simulink model "Ninad_deshpande_Suspensionmodel"  (R2024b)
settings: Solver=ode45  StartTime=0.0  StopTime=10  RelTol=1e-3  EnableMultiTasking=on
values from neighbouring files (symbols this model uses):
  a = 400    [Ninad_deshpande_suspensionscript.m]
  b = 2.5e3    (= 2500)    [Ninad_deshpande_suspensionscript.m]
  Ks = 20e3    (= 20000)    [Ninad_deshpande_suspensionscript.m]
  M_u = 50    [Ninad_deshpande_suspensionscript.m]
settings Model: Creator=lenovo  LastModifiedBy=lenovo
settings SolverCC: AlgebraicLoopSolver=TrustRegion
settings DataIOCC: LimitDataPoints=on  SaveFormat=Array  ReturnWorkspaceOutputs=off
settings OptimizationCC: LifeSpan=inf
settings DebuggingCC: UnconnectedInputMsg=warning  UnconnectedOutputMsg=warning  UnconnectedLineMsg=warning  SFUnexpectedBacktrackingDiag=warning  SFNoUnconditionalDefaultTransitionDiag=warning  SFExecutionAtInitializationDiag=none  ArithmeticOperatorsInVariantConditions=warning
settings HardwareCC: ProdBitPerPointer=32  ProdBitPerSizeT=32  ProdBitPerPtrDiffT=32  ProdLargestAtomicFloat=None  ProdIntDivRoundTo=Undefined  ProdEndianess=Unspecified  ProdWordSize=32  ProdHWDeviceType=32-bit Generic
settings ModelReferenceCC: PropagateSignalLabelsOutOfModel=off
settings SFSimCC: SimUseLocalCustomCode=off  CustomCodeUndefinedFunction=UseInterfaceOnly
settings RTWCC: RTWUseLocalCustomCode=off  GPUComputeCapability=3.5
settings CodeAppCC: StateflowObjectComments=on
settings GRTTargetCC: TargetLangStandard=C89/C90 (ANSI)
settings ConfigComp: CovMetricSettings=dw  CovSaveCumulativeToWorkspaceVar=on  CovSaveSingleToWorkspaceVar=on  CovExternalEMLEnable=off

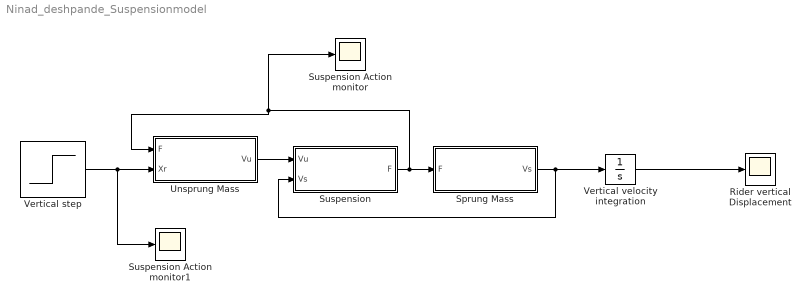
== system Ninad_deshpande_Suspensionmodel ==
  Rider vertical Displacement : Scope
  Sprung Mass : Subsystem
  Suspension : Subsystem
  Suspension Action monitor : Scope
  Suspension Action monitor1 : Scope
  Unsprung Mass : Subsystem
  Vertical step : Step  Time=3  SampleTime=0
  Vertical velocity integration : Integrator
  wires:
  Vertical step/1 -> Suspension Action monitor1/1, Unsprung Mass/2(Xr)
  Unsprung Mass/1(Vu) -> Suspension/1(Vu)
  Suspension/1(F) -> Sprung Mass/1(F), Suspension Action monitor/1, Unsprung Mass/1(F)
  Sprung Mass/1(Vs) -> Suspension/2(Vs), Vertical velocity integration/1
  Vertical velocity integration/1 -> Rider vertical Displacement/1

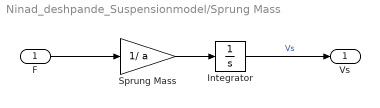
== system Ninad_deshpande_Suspensionmodel/Sprung Mass ==
  F : Inport
  Integrator : Integrator
  Sprung Mass : Gain  Gain=1/ a
  Vs : Outport
  wires:
  Sprung Mass/1 -> Integrator/1
  Integrator/1 -> Vs/1  "Vs"
  F/1 -> Sprung Mass/1

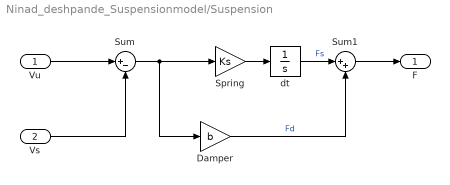
== system Ninad_deshpande_Suspensionmodel/Suspension ==
  Vu : Inport
  Vs : Inport  Port=2
  Damper : Gain  Gain=b
  Spring : Gain  Gain=Ks
  Sum : Sum  Inputs=|+-
  Sum1 : Sum  Inputs=|++
  dt : Integrator
  F : Outport
  wires:
  Sum/1 -> Damper/1, Spring/1
  Vs/1 -> Sum/2
  Vu/1 -> Sum/1
  Sum1/1 -> F/1
  Damper/1 -> Sum1/2  "Fd"
  Spring/1 -> dt/1
  dt/1 -> Sum1/1  "Fs"

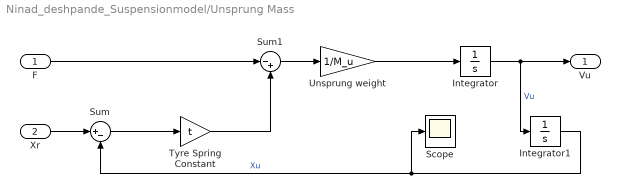
== system Ninad_deshpande_Suspensionmodel/Unsprung Mass ==
  F : Inport
  Xr : Inport  Port=2
  Integrator : Integrator
  Integrator1 : Integrator
  Scope : Scope
  Sum : Sum  Inputs=|+-
  Sum1 : Sum  Inputs=|-+
  Tyre Spring Constant : Gain  Gain=t
  Unsprung weight : Gain  Gain=1/M_u
  Vu : Outport
  wires:
  Xr/1 -> Sum/1
  Sum/1 -> Tyre Spring Constant/1
  F/1 -> Sum1/1
  Tyre Spring Constant/1 -> Sum1/2
  Sum1/1 -> Unsprung weight/1
  Unsprung weight/1 -> Integrator/1
  Integrator/1 -> Integrator1/1, Vu/1  "Vu"
  Integrator1/1 -> Scope/1, Sum/2  "Xu"
